simulink model "SOCPIControlBenchmark"  (R2019b)
settings: Solver=FixedStepAuto  StartTime=0.0  StopTime=30000  FixedStep=0.01  RelTol=1e-3
values from neighbouring files (symbols this model uses):
  kio = 0.6    [benchmarkPIDStart.m]
  kpo = 0.2    [benchmarkPIDStart.m]
  L = 0.1    [benchmarkPIDStart.m]
  maxKi = 0.1    [benchmarkPIDStart.m]
  maxKp = 0.1    [benchmarkPIDStart.m]
  minKi = 0.001    [benchmarkPIDStart.m]
  minKp = 0.01    [benchmarkPIDStart.m]
  N = 100    [benchmarkPIDStart.m]
  optimPeriod = 300    [benchmarkPIDStart.m]
  OVLim = 0.05    [benchmarkPIDStart.m]
  refSignalPeriod = 300    [benchmarkPIDStart.m]
  resetThreshold = 0.1    [benchmarkPIDStart.m]
  TSLim = 70    [benchmarkPIDStart.m]
undefined symbols (not defined in the file or in its folder): DiscIntNeverNeededParam
libraries: dspmathops x4, simulink x2
(part 1 of 3)
settings Model: Creator=jairo  LastModifiedBy=jairo
settings DataIOCC: ReturnWorkspaceOutputs=off

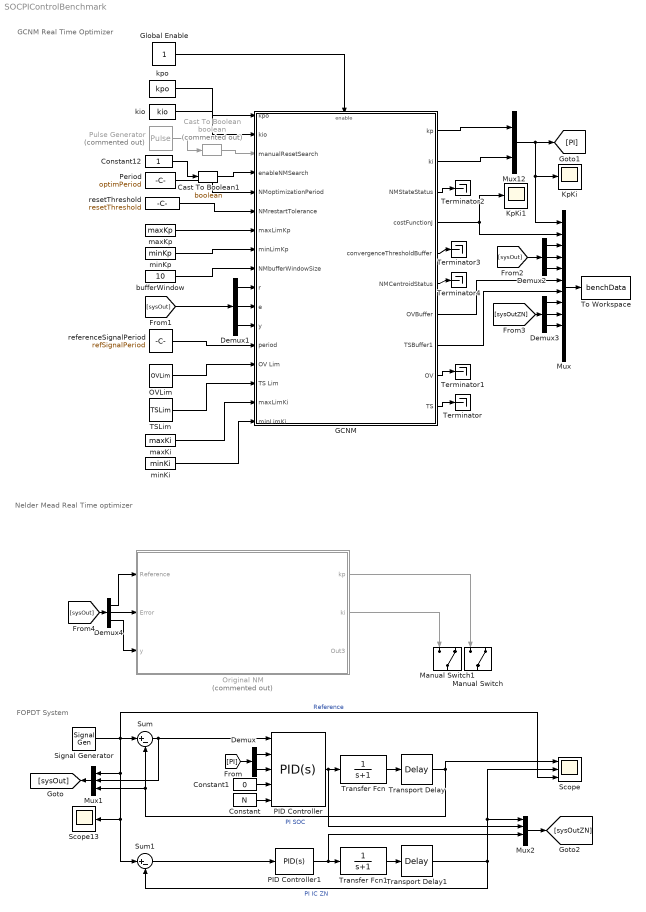
== system SOCPIControlBenchmark ==
  note: FOPDT System
  note: GCNM Real Time Optimizer
  note: Nelder Mead Real Time optimizer
  Cast To Boolean : DataTypeConversion  Commented=on  OutDataTypeStr=boolean
  Cast To Boolean1 : DataTypeConversion  OutDataTypeStr=boolean
  Constant : Constant  Value=N
  Constant1 : Constant  Value=0
  Constant12 : Constant  OutDataTypeStr=boolean
  Demux : Demux  Outputs=2
  Demux{1..4} (4 alike) : Demux  Outputs=3
  GCNM : Subsystem
  Global Enable : Constant
  KpKi : Scope
  KpKi1 : Scope
  Manual Switch : ManualSwitch  CurrentSetting=0
  Manual Switch1 : ManualSwitch  CurrentSetting=0
  Mux : Mux  Inputs=12
  Mux1 : Mux  Inputs=3
  Mux12 : Mux  Inputs=2
  Mux2 : Mux
  OVLim : Constant  Value=OVLim
  Original NM : Subsystem  Commented=on
  PID Controller : simulink/Continuous/PID Controller  Controller=PID  Form=Parallel  TimeDomain=Continuous-time  SampleTime=-1  IntegratorMethod=Forward Euler  FilterMethod=Forward Euler  ControllerParametersSource=external  P=1  I=100  D=0  UseFilter=on  N=100  TunerSelectOption=Transfer Function Based (PID Tuner App)  InitialConditionSource=internal  InitialConditionForIntegrator=0  InitialConditionForFilter=0  DifferentiatorICPrevScaledInput=0  ExternalReset=none  TrackingMode=off  Kt=1  LimitOutput=off  UpperSaturationLimit=inf  LowerSaturationLimit=-inf  LinearizeAsGain=on  AntiWindupMode=none  Kb=1  POutMin=[]  POutMax=[]  IOutMin=[]  IOutMax=[]  DOutMin=[]  DOutMax=[]  NOutMin=[]  NOutMax=[]  SumOutMin=[]  SumOutMax=[]  SaturationOutMin=[]  SaturationOutMax=[]  PParamMin=[]  PParamMax=[]  IParamMin=[]  IParamMax=[]  DParamMin=[]  DParamMax=[]  NParamMin=[]  NParamMax=[]  KbParamMin=[]  KbParamMax=[]  KtParamMin=[]  KtParamMax=[]  KbOutMin=[]  KbOutMax=[]  KtOutMin=[]  KtOutMax=[]  IntegratorOutMin=[]  IntegratorOutMax=[]  FilterOutMin=[]  FilterOutMax=[]  SumI1OutMin=[]  SumI1OutMax=[]  SumI2OutMin=[]  SumI2OutMax=[]  SumI3OutMin=[]  SumI3OutMax=[]  SumI4OutMin=[]  SumI4OutMax=[]  SumDOutMin=[]  SumDOutMax=[]  DifferentiatorOutMin=[]  DifferentiatorOutMax=[]  FilterDiffOutCoefMin=[]  FilterDiffOutCoefMax=[]  ReciprocalOutMin=[]  ReciprocalOutMax=[]  SumDenOutMin=[]  SumDenOutMax=[]  SumNumOutMin=[]  SumNumOutMax=[]  DivideOutMin=[]  DivideOutMax=[]  IntegratorContinuousStateAttributes=''  IntegratorStateMustResolveToSignalObject=off  IntegratorRTWStateStorageClass=Auto  FilterContinuousStateAttributes=''  FilterStateMustResolveToSignalObject=off  FilterRTWStateStorageClass=Auto  ParallelPVariant=ExternalParameters  IdealPVariant=Disabled  IVariant=ExternalParameters  DVariant=ExternalParameters  IntegratorVariant=Continuous  SatVariant=Disabled  AWVariant=Passthrough  PCopyVariant=Disabled  TRVariant=Disabled  FdbkBlocksVariant=Forward  IdealPFdbkVariant=Disabled  SatFdbkVariant=Disabled  DerivativeFilterVariant=ContFilter  NVariant=ExternalParameters  NCopyVariant=Disabled  FilterICVariant=InternalICsFilter  IntegratorICVariant=InternalICs  ExternalResetVariant=Disabled  TRSumVariant=Passthrough  SumFdbkVariant=Disabled  SumVariant=Sum_PID
  PID Controller1 : simulink/Continuous/PID Controller  Controller=PID  Form=Parallel  TimeDomain=Continuous-time  SampleTime=-1  IntegratorMethod=Forward Euler  FilterMethod=Forward Euler  ControllerParametersSource=internal  P=.12  I=0.006  D=0  UseFilter=on  N=100  TunerSelectOption=Transfer Function Based (PID Tuner App)  InitialConditionSource=internal  InitialConditionForIntegrator=0  InitialConditionForFilter=0  DifferentiatorICPrevScaledInput=0  ExternalReset=none  TrackingMode=off  Kt=1  LimitOutput=off  UpperSaturationLimit=inf  LowerSaturationLimit=-inf  LinearizeAsGain=on  AntiWindupMode=none  Kb=1  POutMin=[]  POutMax=[]  IOutMin=[]  IOutMax=[]  DOutMin=[]  DOutMax=[]  NOutMin=[]  NOutMax=[]  SumOutMin=[]  SumOutMax=[]  SaturationOutMin=[]  SaturationOutMax=[]  PParamMin=[]  PParamMax=[]  IParamMin=[]  IParamMax=[]  DParamMin=[]  DParamMax=[]  NParamMin=[]  NParamMax=[]  KbParamMin=[]  KbParamMax=[]  KtParamMin=[]  KtParamMax=[]  KbOutMin=[]  KbOutMax=[]  KtOutMin=[]  KtOutMax=[]  IntegratorOutMin=[]  IntegratorOutMax=[]  FilterOutMin=[]  FilterOutMax=[]  SumI1OutMin=[]  SumI1OutMax=[]  SumI2OutMin=[]  SumI2OutMax=[]  SumI3OutMin=[]  SumI3OutMax=[]  SumI4OutMin=[]  SumI4OutMax=[]  SumDOutMin=[]  SumDOutMax=[]  DifferentiatorOutMin=[]  DifferentiatorOutMax=[]  FilterDiffOutCoefMin=[]  FilterDiffOutCoefMax=[]  ReciprocalOutMin=[]  ReciprocalOutMax=[]  SumDenOutMin=[]  SumDenOutMax=[]  SumNumOutMin=[]  SumNumOutMax=[]  DivideOutMin=[]  DivideOutMax=[]  IntegratorContinuousStateAttributes=''  IntegratorStateMustResolveToSignalObject=off  IntegratorRTWStateStorageClass=Auto  FilterContinuousStateAttributes=''  FilterStateMustResolveToSignalObject=off  FilterRTWStateStorageClass=Auto  ParallelPVariant=InternalParameters  IdealPVariant=Disabled  IVariant=InternalParameters  DVariant=InternalParameters  IntegratorVariant=Continuous  SatVariant=Disabled  AWVariant=Passthrough  PCopyVariant=Disabled  TRVariant=Disabled  FdbkBlocksVariant=Forward  IdealPFdbkVariant=Disabled  SatFdbkVariant=Disabled  DerivativeFilterVariant=ContFilter  NVariant=InternalParameters  NCopyVariant=Disabled  FilterICVariant=InternalICsFilter  IntegratorICVariant=InternalICs  ExternalResetVariant=Disabled  TRSumVariant=Passthrough  SumFdbkVariant=Disabled  SumVariant=Sum_PID
  Period : Constant  Value=optimPeriod  OutDataTypeStr=double
  Pulse Generator : DiscretePulseGenerator  Commented=on  PulseType=Time based  Period=20  PulseWidth=0.1
  Scope : Scope  NumInputPorts=3
  Scope13 : Scope
  Signal Generator : SignalGenerator  WaveForm=square  Frequency=1/refSignalPeriod
  Sum : Sum  Inputs=|+-
  Sum1 : Sum  Inputs=|+-
  TSLim : Constant  Value=TSLim
  Terminator{,1..4} (5 alike) : Terminator
  To Workspace : ToWorkspace  VariableName=benchData  SaveFormat=Timeseries  SampleTime=-1
  Transfer Fcn : TransferFcn  Denominator=[1 1]
  Transfer Fcn1 : TransferFcn  Denominator=[1 1]
  Transport Delay : TransportDelay  DelayTime=L
  Transport Delay1 : TransportDelay  DelayTime=L
  bufferWindow : Constant  Value=10  OutDataTypeStr=uint16
  kio : Constant  Value=kio  OutDataTypeStr=double
  kpo : Constant  Value=kpo  OutDataTypeStr=double
  maxKi : Constant  Value=maxKi  VectorParams1D=off  OutDataTypeStr=double
  maxKp : Constant  Value=maxKp  OutDataTypeStr=double
  minKi : Constant  Value=minKi  OutDataTypeStr=double
  minKp : Constant  Value=minKp  OutDataTypeStr=double
  referenceSignalPeriod : Constant  Value=refSignalPeriod
  resetThreshold : Constant  Value=resetThreshold
  wires:
  PID Controller/1 -> Mux2/2, Transfer Fcn/1
  Transfer Fcn/1 -> Transport Delay/1
  Transfer Fcn1/1 -> Transport Delay1/1
  Sum1/1 -> PID Controller1/1
  PID Controller1/1 -> Mux2/3, Transfer Fcn1/1
  Sum/1 -> Mux1/2, PID Controller/1
  resetThreshold/1 -> GCNM/6(NMrestartTolerance)
  Mux12/1 -> Mux/1, KpKi/1, [PI]
  maxKp/1 -> GCNM/7(maxLimKp)
  bufferWindow/1 -> GCNM/9(NMbufferWindowSize)
  Cast To Boolean1/1 -> GCNM/4(enableNMSearch)
  kio/1 -> GCNM/2(kio)
  Pulse Generator/1 -> Cast To Boolean/1
  Cast To Boolean/1 -> GCNM/3(manualResetSearch)
  Constant12/1 -> Cast To Boolean1/1
  minKp/1 -> GCNM/8(minLimKp)
  Global Enable/1 -> GCNM/Enable
  kpo/1 -> GCNM/1(kpo)
  Period/1 -> GCNM/5(NMoptimizationPeriod)
  GCNM/4(costFunctionJ) -> Mux/2, KpKi1/1
  referenceSignalPeriod/1 -> GCNM/13("  period")
  OVLim/1 -> GCNM/14("  OV Lim")
  TSLim/1 -> GCNM/15(TS Lim)
  Transport Delay/1 -> Scope/1, Mux1/3, Sum/2  "PI SOC"
  Transport Delay1/1 -> Mux2/1, Scope/2, Sum1/2  "PI IC ZN"
  GCNM/1("  kp") -> Mux12/1
  GCNM/2("  ki") -> Mux12/2
  Original NM/1(kp) -> Manual Switch/1
  Original NM/2(ki) -> Manual Switch1/1
  Mux/1 -> To Workspace/1
  maxKi/1 -> GCNM/16(maxLimKi)
  minKi/1 -> GCNM/17(minLimKi)
  Constant/1 -> PID Controller/5
  Signal Generator/1 -> Sum1/1, Scope13/1, Mux1/1, Scope/3, Sum/1  "Reference"
  Constant1/1 -> PID Controller/4
  Demux/1 -> PID Controller/2
  Demux/2 -> PID Controller/3
  [PI] -> Demux/1
  Mux1/1 -> [sysOut]
  [sysOut] -> Demux1/1
  Demux1/1 -> GCNM/10("  r")
  Demux1/2 -> GCNM/11("  e")
  Demux1/3 -> GCNM/12("  y")
  [sysOut] -> Demux2/1
  Demux2/1 -> Mux/3
  Demux2/2 -> Mux/4
  Demux2/3 -> Mux/5
  Mux2/1 -> [sysOutZN]
  [sysOutZN] -> Demux3/1
  Demux3/1 -> Mux/8
  Demux3/2 -> Mux/9
  Demux3/3 -> Mux/10
  Demux4/2 -> Original NM/2(Error)
  Demux4/3 -> Original NM/3(y)
  [sysOut] -> Demux4/1
  Demux4/1 -> Original NM/1(Reference)
  GCNM/10(TS) -> Terminator/1
  GCNM/9(OV) -> Terminator1/1
  GCNM/8(TSBuffer1) -> Mux/7
  GCNM/7(OVBuffer) -> Mux/6
  GCNM/3(NMStateStatus) -> Terminator2/1
  GCNM/5(convergenceThresholdBuffer) -> Terminator3/1
  GCNM/6(NMCentroidStatus) -> Terminator4/1

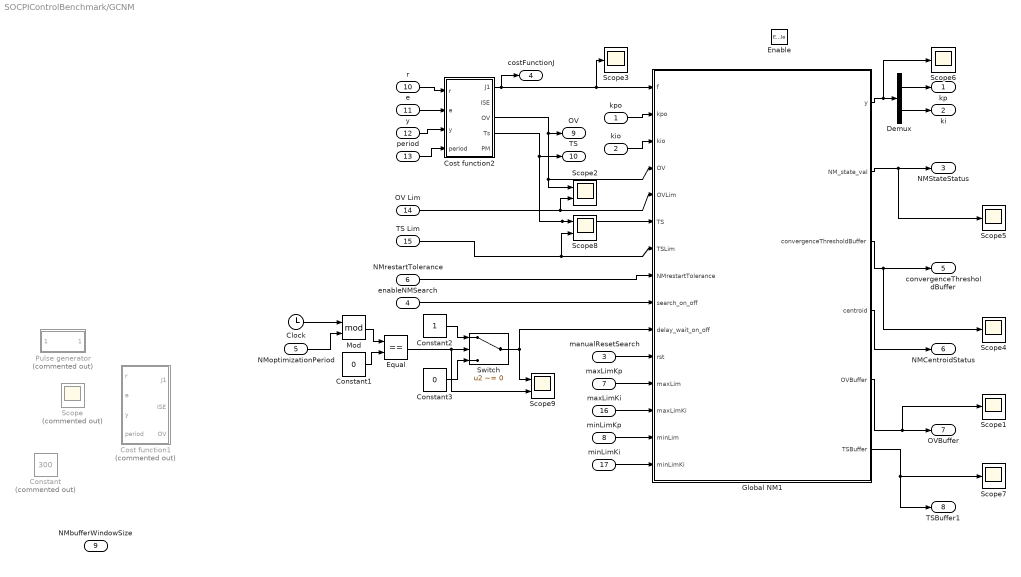
== system SOCPIControlBenchmark/GCNM ==
  kpo : Inport  OutDataTypeStr=double
  kio : Inport  Port=2  OutDataTypeStr=double
  manualResetSearch : Inport  Port=3  OutDataTypeStr=boolean
  enableNMSearch : Inport  Port=4  OutDataTypeStr=boolean
  NMoptimizationPeriod : Inport  Port=5  OutDataTypeStr=double
  NMrestartTolerance : Inport  Port=6
  maxLimKp : Inport  Port=7  OutDataTypeStr=double
  minLimKp : Inport  Port=8  OutDataTypeStr=double
  NMbufferWindowSize : Inport  Port=9  OutDataTypeStr=uint16
  "  r" : Inport  Port=10  OutDataTypeStr=double
  "  e" : Inport  Port=11  OutDataTypeStr=double
  "  y" : Inport  Port=12  OutDataTypeStr=double
  "  period" : Inport  Port=13  OutDataTypeStr=double
  "  OV Lim" : Inport  Port=14  OutDataTypeStr=double
  TS Lim : Inport  Port=15  OutDataTypeStr=double
  maxLimKi : Inport  Port=16  OutDataTypeStr=double
  minLimKi : Inport  Port=17  OutDataTypeStr=double
  Enable : EnablePort
  Clock : Clock
  Constant : Constant  Commented=on  Value=300
  Constant1 : Constant  Value=0
  Constant2 : Constant
  Constant3 : Constant  Value=0
  Cost function1 : Subsystem  Commented=on
  Cost function2 : Subsystem
  Demux : Demux  Outputs=2
  Equal : RelationalOperator  Operator===  RndMeth=Simplest
  Global NM1 : MATLAB Function  TreatAsAtomicUnit=on
  Mod : Math  Operator=mod  SignedPower=off  SaturateOnIntegerOverflow=on
  Pulse generator : Subsystem  Commented=on
  Scope : Scope  Commented=on
  Scope{1,3..7} (6 alike) : Scope
  Scope2 : Scope  NumInputPorts=2
  Scope8 : Scope  NumInputPorts=2
  Scope9 : Scope  NumInputPorts=2
  Switch : Switch  Criteria=u2 ~= 0
  "  kp" : Outport  OutDataTypeStr=double
  "  ki" : Outport  Port=2  OutDataTypeStr=double
  NMStateStatus : Outport  Port=3  OutDataTypeStr=double
  costFunctionJ : Outport  Port=4  OutDataTypeStr=double
  convergenceThresholdBuffer : Outport  Port=5  OutDataTypeStr=double
  NMCentroidStatus : Outport  Port=6  OutDataTypeStr=double
  OVBuffer : Outport  Port=7  OutDataTypeStr=double
  TSBuffer1 : Outport  Port=8  OutDataTypeStr=double
  OV : Outport  Port=9  OutDataTypeStr=double
  TS : Outport  Port=10  OutDataTypeStr=double
  wires:
  Demux/2 -> "  ki"/1
  Demux/1 -> "  kp"/1
  NMrestartTolerance/1 -> Global NM1/8(NMrestartTolerance)
  manualResetSearch/1 -> Global NM1/11(rst)
  enableNMSearch/1 -> Global NM1/9(search_on_off)
  minLimKp/1 -> Global NM1/14(minLim)
  maxLimKp/1 -> Global NM1/12(maxLim)
  Global NM1/2(NM_state_val) -> Scope5/1, NMStateStatus/1
  Global NM1/3(convergenceThresholdBuffer) -> convergenceThresholdBuffer/1, Scope4/1
  Global NM1/4(centroid) -> NMCentroidStatus/1
  Global NM1/1(y) -> Scope6/1, Demux/1
  kpo/1 -> Global NM1/2(kpo)
  kio/1 -> Global NM1/3(kio)
  Cost function2/3(OV) -> OV/1, Global NM1/4(OV), Scope2/1
  "  y"/1 -> Cost function2/3(y)
  "  e"/1 -> Cost function2/2(e)
  "  r"/1 -> Cost function2/1(r)
  Global NM1/5(OVBuffer) -> Scope1/1, OVBuffer/1
  "  period"/1 -> Cost function2/4(period)
  "  OV Lim"/1 -> Scope2/2, Global NM1/5(OVLim)
  Cost function2/4(Ts) -> TS/1, Global NM1/6(TS), Scope8/1
  TS Lim/1 -> Scope8/2, Global NM1/7(TSLim)
  Global NM1/6(TSBuffer) -> TSBuffer1/1, Scope7/1
  Cost function2/1(J1) -> Scope3/1, Global NM1/1(f), costFunctionJ/1
  Clock/1 -> Mod/1
  NMoptimizationPeriod/1 -> Mod/2
  Constant1/1 -> Equal/2
  Mod/1 -> Equal/1
  Constant2/1 -> Switch/1
  Constant3/1 -> Switch/3
  Switch/1 -> Scope9/1, Global NM1/10(delay_wait_on_off)
  Equal/1 -> Scope9/2, Switch/2
  maxLimKi/1 -> Global NM1/13(maxLimKi)
  minLimKi/1 -> Global NM1/15(minLimKi)

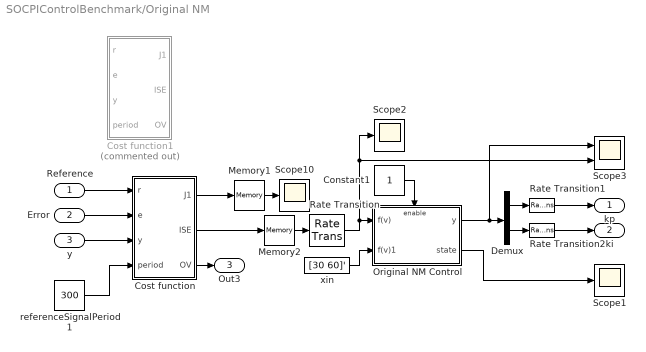
== system SOCPIControlBenchmark/Original NM ==
  Reference : Inport
  Error : Inport  Port=2
  y : Inport  Port=3
  Constant1 : Constant
  Cost function : Subsystem
  Cost function1 : Subsystem  Commented=on
  Demux : Demux  Outputs=2
  Memory1 : Memory
  Memory2 : Memory
  Original NM Control : Subsystem
  Rate Transition : RateTransition
  Rate Transition1 : RateTransition  InitialCondition=1
  Rate Transition2 : RateTransition  InitialCondition=100
  Scope1 : Scope
  Scope10 : Scope
  Scope2 : Scope
  Scope3 : Scope  NumInputPorts=2
  referenceSignalPeriod1 : Constant  Value=300
  xin : Constant  Value=[30 60]'
  kp : Outport
  ki : Outport  Port=2
  Out3 : Outport  Port=3
  wires:
  Constant1/1 -> Original NM Control/Enable
  Original NM Control/1(y) -> Scope3/1, Demux/1
  Rate Transition/1 -> Scope2/1, Scope3/2, Original NM Control/1(f(v))
  Demux/2 -> Rate Transition2/1
  xin/1 -> Original NM Control/2(f(v)1)
  y/1 -> Cost function/3(y)
  Original NM Control/2(state) -> Scope1/1
  Demux/1 -> Rate Transition1/1
  Memory2/1 -> Rate Transition/1
  Cost function/3(OV) -> Out3/1
  Memory1/1 -> Scope10/1
  referenceSignalPeriod1/1 -> Cost function/4(period)
  Cost function/1(J1) -> Memory1/1
  Cost function/2(ISE) -> Memory2/1
  Rate Transition1/1 -> kp/1
  Rate Transition2/1 -> ki/1
  Reference/1 -> Cost function/1(r)
  Error/1 -> Cost function/2(e)

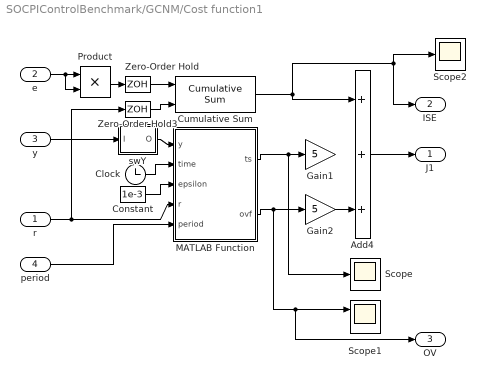
== system SOCPIControlBenchmark/GCNM/Cost function1 ==
  r : Inport
  e : Inport  Port=2
  y : Inport  Port=3
  period : Inport  Port=4
  Add4 : Sum  Inputs=+++
  Clock : Clock
  Constant : Constant  Value=1e-3
  Cumulative Sum : dspmathops/Cumulative Sum  dim=Channels (running sum)  InputProcessing=Columns as channels (frame based)  reset_popup=Falling edge  roundingMode=Floor  overflowMode=off  outputDataTypeStr=Inherit: Same as accumulator  outputMin=[]  outputMax=[]  outputLastDataTypeStr=Inherit: Same as accumulator
      settings: SourceProductName=DSP System Toolbox
  Gain1 : Gain  Gain=5
  Gain2 : Gain  Gain=5
  MATLAB Function : MATLAB Function  TreatAsAtomicUnit=on
  Product : Product
  Scope : Scope
  Scope1 : Scope  NumInputPorts=2
  Scope2 : Scope
  Zero-Order Hold : ZeroOrderHold  SampleTime=-1
  Zero-Order Hold3 : ZeroOrderHold  SampleTime=-1
  swY : Subsystem
  J1 : Outport
  ISE : Outport  Port=2
  OV : Outport  Port=3
  wires:
  period/1 -> MATLAB Function/5(period)
  Gain2/1 -> Add4/3
  Add4/1 -> J1/1
  y/1 -> swY/1(I)
  Constant/1 -> MATLAB Function/3(epsilon)
  Product/1 -> Zero-Order Hold/1
  Clock/1 -> MATLAB Function/2(time)
  swY/1(O) -> MATLAB Function/1(y)
  MATLAB Function/2(ovf) -> Gain2/1, Scope1/1, OV/1
  r/1 -> MATLAB Function/4(r), Zero-Order Hold3/1
  Zero-Order Hold/1 -> Cumulative Sum/1
  MATLAB Function/1(ts) -> Gain1/1, Scope/1
  e/1 -> Product/1, Product/2
  Zero-Order Hold3/1 -> Cumulative Sum/2
  Cumulative Sum/1 -> Scope2/1, ISE/1, Add4/1

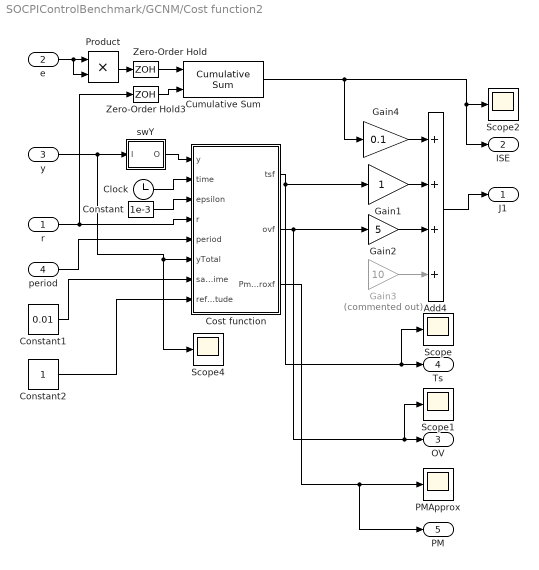
== system SOCPIControlBenchmark/GCNM/Cost function2 ==
  r : Inport
  e : Inport  Port=2
  y : Inport  Port=3
  period : Inport  Port=4
  Add4 : Sum  Inputs=++++
  Clock : Clock
  Constant : Constant  Value=1e-3
  Constant1 : Constant  Value=0.01
  Constant2 : Constant
  Cost function : MATLAB Function  TreatAsAtomicUnit=on
  Cumulative Sum : dspmathops/Cumulative Sum  dim=Channels (running sum)  InputProcessing=Columns as channels (frame based)  reset_popup=Falling edge  roundingMode=Floor  overflowMode=off  outputDataTypeStr=Inherit: Same as accumulator  outputMin=[]  outputMax=[]  outputLastDataTypeStr=Inherit: Same as accumulator
      settings: SourceProductName=DSP System Toolbox
  Gain1 : Gain
  Gain2 : Gain  Gain=5
  Gain3 : Gain  Commented=on  Gain=10
  Gain4 : Gain  Gain=0.1
  PMApprox : Scope
  Product : Product
  Scope{,1..2,4} (4 alike) : Scope
  Zero-Order Hold : ZeroOrderHold  SampleTime=-1
  Zero-Order Hold3 : ZeroOrderHold  SampleTime=-1
  swY : Subsystem
  J1 : Outport
  ISE : Outport  Port=2
  OV : Outport  Port=3
  Ts : Outport  Port=4
  PM : Outport  Port=5
  wires:
  Cumulative Sum/1 -> Gain4/1, ISE/1, Scope2/1
  Zero-Order Hold3/1 -> Cumulative Sum/2
  e/1 -> Product/2, Product/1
  Zero-Order Hold/1 -> Cumulative Sum/1
  r/1 -> Zero-Order Hold3/1, Cost function/4(r)
  swY/1(O) -> Cost function/1(y)
  Clock/1 -> Cost function/2(time)
  Product/1 -> Zero-Order Hold/1
  Constant/1 -> Cost function/3(epsilon)
  y/1 -> Scope4/1, Cost function/6(yTotal), swY/1(I)
  Add4/1 -> J1/1
  Gain2/1 -> Add4/3
  period/1 -> Cost function/5(period)
  Constant1/1 -> Cost function/7(samplingTime)
  Gain1/1 -> Add4/2
  Constant2/1 -> Cost function/8(refAmplitude)
  Gain3/1 -> Add4/4
  Cost function/1(tsf) -> Scope/1, Ts/1, Gain1/1
  Cost function/2(ovf) -> Scope1/1, OV/1, Gain2/1
  Cost function/3(PmAproxf) -> PM/1, PMApprox/1
  Gain4/1 -> Add4/1

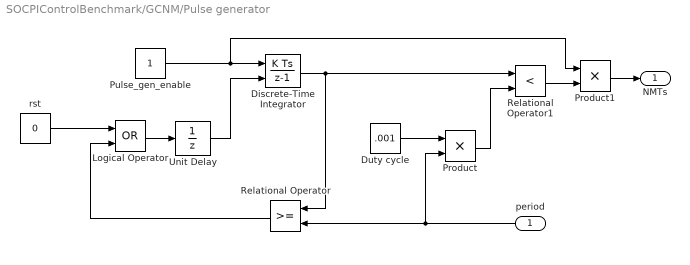
== system SOCPIControlBenchmark/GCNM/Pulse generator ==
  period : Inport
  Discrete-Time Integrator : DiscreteIntegrator  ExternalReset=rising  SampleTime=-1  ICPrevOutput=DiscIntNeverNeededParam  ICPrevScaledInput=DiscIntNeverNeededParam
  Duty cycle : Constant  Value=.001
  Logical Operator : Logic  Operator=OR  AllPortsSameDT=off  OutDataTypeStr=boolean
  Product : Product  RndMeth=Zero
  Product1 : Product  RndMeth=Zero
  Pulse_gen_enable : Constant
  Relational Operator : RelationalOperator  OutDataTypeStr=boolean  RndMeth=Nearest
  Relational Operator1 : RelationalOperator  Operator=<  OutDataTypeStr=boolean  RndMeth=Nearest
  Unit Delay : UnitDelay  SampleTime=-1
  rst : Constant  Value=0
  NMTs : Outport
  wires:
  Pulse_gen_enable/1 -> Discrete-Time Integrator/1, Product1/1
  Unit Delay/1 -> Discrete-Time Integrator/2
  Duty cycle/1 -> Product/1
  Product/1 -> Relational Operator1/2
  Discrete-Time Integrator/1 -> Relational Operator/1, Relational Operator1/1
  period/1 -> Relational Operator/2, Product/2
  Logical Operator/1 -> Unit Delay/1
  rst/1 -> Logical Operator/1
  Relational Operator/1 -> Logical Operator/2
  Relational Operator1/1 -> Product1/2
  Product1/1 -> NMTs/1

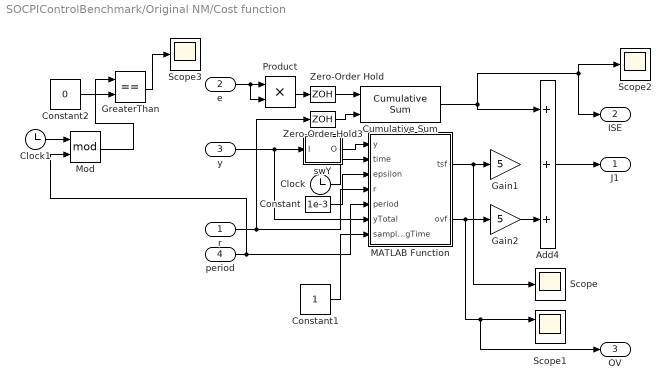
== system SOCPIControlBenchmark/Original NM/Cost function ==
  r : Inport
  e : Inport  Port=2
  y : Inport  Port=3
  period : Inport  Port=4
  Add4 : Sum  Inputs=+++
  Clock : Clock
  Clock1 : Clock
  Constant : Constant  Value=1e-3
  Constant1 : Constant
  Constant2 : Constant  Value=0
  Cumulative Sum : dspmathops/Cumulative Sum  dim=Channels (running sum)  InputProcessing=Columns as channels (frame based)  reset_popup=Falling edge  roundingMode=Floor  overflowMode=off  outputDataTypeStr=Inherit: Same as accumulator  outputMin=[]  outputMax=[]  outputLastDataTypeStr=Inherit: Same as accumulator
      settings: SourceProductName=DSP System Toolbox
  Gain1 : Gain  Gain=5
  Gain2 : Gain  Gain=5
  GreaterThan : RelationalOperator  Operator===  OutDataTypeStr=boolean  RndMeth=Simplest
  MATLAB Function : MATLAB Function  TreatAsAtomicUnit=on
  Mod : Math  Operator=mod  SignedPower=off  SaturateOnIntegerOverflow=on
  Product : Product
  Scope : Scope
  Scope1 : Scope  NumInputPorts=2
  Scope2 : Scope
  Scope3 : Scope
  Zero-Order Hold : ZeroOrderHold  SampleTime=-1
  Zero-Order Hold3 : ZeroOrderHold  SampleTime=-1
  swY : Subsystem
  J1 : Outport
  ISE : Outport  Port=2
  OV : Outport  Port=3
  wires:
  Cumulative Sum/1 -> Add4/1, ISE/1, Scope2/1
  Zero-Order Hold3/1 -> Cumulative Sum/2
  e/1 -> Product/2, Product/1
  MATLAB Function/1(tsf) -> Scope/1, Gain1/1
  Zero-Order Hold/1 -> Cumulative Sum/1
  r/1 -> Zero-Order Hold3/1, MATLAB Function/4(r)
  MATLAB Function/2(ovf) -> OV/1, Scope1/1, Gain2/1
  swY/1(O) -> MATLAB Function/1(y)
  Clock/1 -> MATLAB Function/2(time)
  Product/1 -> Zero-Order Hold/1
  Constant/1 -> MATLAB Function/3(epsilon)
  y/1 -> MATLAB Function/6(yTotal), swY/1(I)
  Add4/1 -> J1/1
  Gain2/1 -> Add4/3
  Constant1/1 -> MATLAB Function/7(samplingTime)
  Clock1/1 -> Mod/1
  Mod/1 -> GreaterThan/1
  period/1 -> MATLAB Function/5(period), Mod/2
  GreaterThan/1 -> Scope3/1
  Constant2/1 -> GreaterThan/2

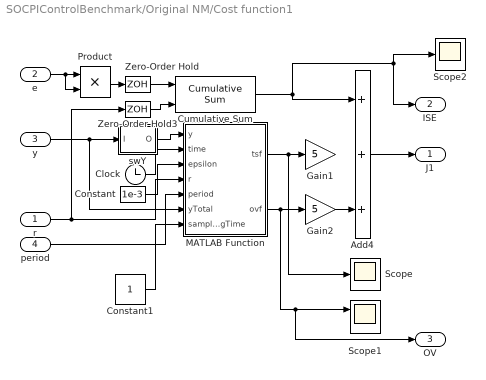
== system SOCPIControlBenchmark/Original NM/Cost function1 ==
  r : Inport
  e : Inport  Port=2
  y : Inport  Port=3
  period : Inport  Port=4
  Add4 : Sum  Inputs=+++
  Clock : Clock
  Constant : Constant  Value=1e-3
  Constant1 : Constant
  Cumulative Sum : dspmathops/Cumulative Sum  dim=Channels (running sum)  InputProcessing=Columns as channels (frame based)  reset_popup=Falling edge  roundingMode=Floor  overflowMode=off  outputDataTypeStr=Inherit: Same as accumulator  outputMin=[]  outputMax=[]  outputLastDataTypeStr=Inherit: Same as accumulator
      settings: SourceProductName=DSP System Toolbox
  Gain1 : Gain  Gain=5
  Gain2 : Gain  Gain=5
  MATLAB Function : MATLAB Function  TreatAsAtomicUnit=on
  Product : Product
  Scope : Scope
  Scope1 : Scope  NumInputPorts=2
  Scope2 : Scope
  Zero-Order Hold : ZeroOrderHold  SampleTime=-1
  Zero-Order Hold3 : ZeroOrderHold  SampleTime=-1
  swY : Subsystem
  J1 : Outport
  ISE : Outport  Port=2
  OV : Outport  Port=3
  wires:
  Constant1/1 -> MATLAB Function/7(samplingTime)
  period/1 -> MATLAB Function/5(period)
  Gain2/1 -> Add4/3
  Add4/1 -> J1/1
  y/1 -> swY/1(I), MATLAB Function/6(yTotal)
  Constant/1 -> MATLAB Function/3(epsilon)
  Product/1 -> Zero-Order Hold/1
  Clock/1 -> MATLAB Function/2(time)
  swY/1(O) -> MATLAB Function/1(y)
  MATLAB Function/2(ovf) -> Gain2/1, Scope1/1, OV/1
  r/1 -> MATLAB Function/4(r), Zero-Order Hold3/1
  Zero-Order Hold/1 -> Cumulative Sum/1
  MATLAB Function/1(tsf) -> Gain1/1, Scope/1
  e/1 -> Product/1, Product/2
  Zero-Order Hold3/1 -> Cumulative Sum/2
  Cumulative Sum/1 -> Scope2/1, ISE/1, Add4/1

== system SOCPIControlBenchmark/Original NM/Original NM Control ==
  note: Official backups
  f(v) : Inport
  f(v)1 : Inport  Port=2
  Enable : EnablePort
  Global NM : MATLAB Function  Commented=on  TreatAsAtomicUnit=on
  Original NM : MATLAB Function  Commented=on  TreatAsAtomicUnit=on
  Original NM2 : MATLAB Function  TreatAsAtomicUnit=on  SystemSampleTime=10
  Scope : Scope
  y : Outport
  state : Outport  Port=2
  wires:
  f(v)/1 -> Scope/1, Original NM2/1(f)
  Original NM2/1(y) -> y/1
  Original NM2/2(NM_state_val) -> state/1
  f(v)1/1 -> Original NM2/2(x)

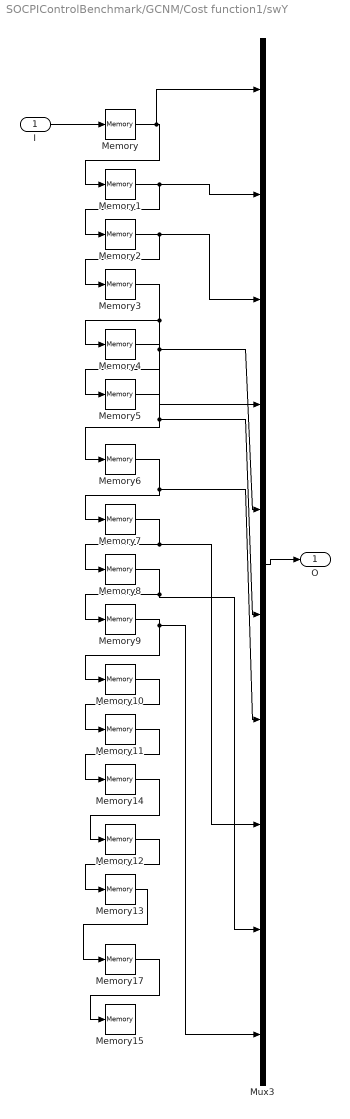
== system SOCPIControlBenchmark/GCNM/Cost function1/swY ==
  I : Inport
  Memory{,1..15,17} (17 alike) : Memory
  Mux3 : Mux  Inputs=10
  O : Outport
  wires:
  Memory17/1 -> Memory15/1
  Memory7/1 -> Mux3/8, Memory8/1
  Memory/1 -> Mux3/1, Memory1/1
  Memory8/1 -> Mux3/9, Memory9/1
  I/1 -> Memory/1
  Memory2/1 -> Mux3/3, Memory3/1
  Memory10/1 -> Memory11/1
  Memory1/1 -> Mux3/2, Memory2/1
  Memory6/1 -> Mux3/7, Memory7/1
  Memory3/1 -> Mux3/4, Memory4/1
  Memory9/1 -> Mux3/10, Memory10/1
  Mux3/1 -> O/1
  Memory4/1 -> Mux3/5, Memory5/1
  Memory5/1 -> Mux3/6, Memory6/1
  Memory13/1 -> Memory17/1
  Memory12/1 -> Memory13/1
  Memory14/1 -> Memory12/1
  Memory11/1 -> Memory14/1

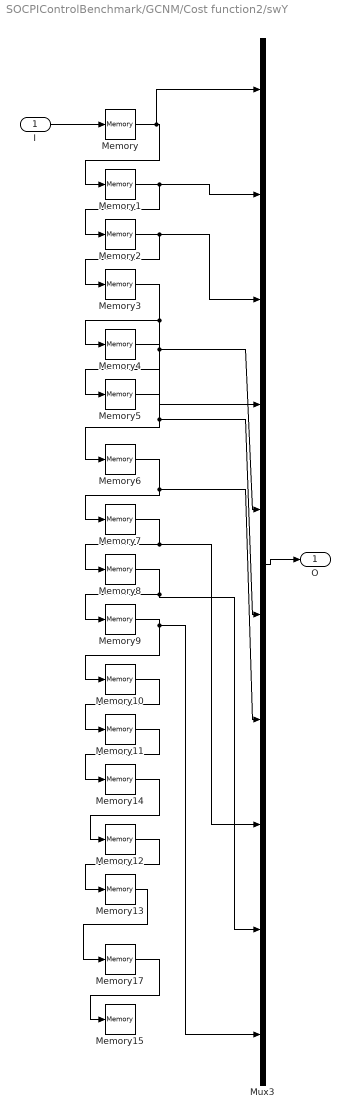
== system SOCPIControlBenchmark/GCNM/Cost function2/swY ==
  I : Inport
  Memory{,1..15,17} (17 alike) : Memory
  Mux3 : Mux  Inputs=10
  O : Outport
  wires:
  Memory11/1 -> Memory14/1
  Memory14/1 -> Memory12/1
  Memory12/1 -> Memory13/1
  Memory13/1 -> Memory17/1
  Memory5/1 -> Memory6/1, Mux3/6
  Memory4/1 -> Memory5/1, Mux3/5
  Mux3/1 -> O/1
  Memory9/1 -> Memory10/1, Mux3/10
  Memory3/1 -> Memory4/1, Mux3/4
  Memory6/1 -> Memory7/1, Mux3/7
  Memory1/1 -> Memory2/1, Mux3/2
  Memory10/1 -> Memory11/1
  Memory2/1 -> Memory3/1, Mux3/3
  I/1 -> Memory/1
  Memory8/1 -> Memory9/1, Mux3/9
  Memory/1 -> Memory1/1, Mux3/1
  Memory7/1 -> Memory8/1, Mux3/8
  Memory17/1 -> Memory15/1

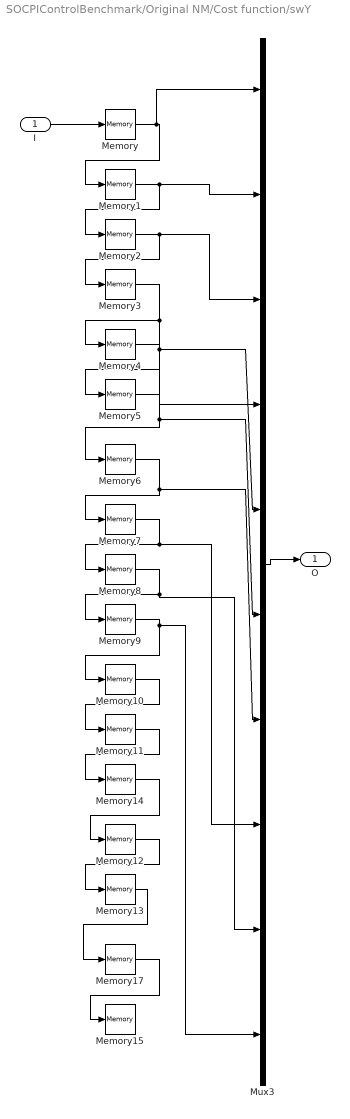
== system SOCPIControlBenchmark/Original NM/Cost function/swY ==
  I : Inport
  Memory{,1..15,17} (17 alike) : Memory
  Mux3 : Mux  Inputs=10
  O : Outport
  wires:
  Memory11/1 -> Memory14/1
  Memory14/1 -> Memory12/1
  Memory12/1 -> Memory13/1
  Memory13/1 -> Memory17/1
  Memory5/1 -> Memory6/1, Mux3/6
  Memory4/1 -> Memory5/1, Mux3/5
  Mux3/1 -> O/1
  Memory9/1 -> Memory10/1, Mux3/10
  Memory3/1 -> Memory4/1, Mux3/4
  Memory6/1 -> Memory7/1, Mux3/7
  Memory1/1 -> Memory2/1, Mux3/2
  Memory10/1 -> Memory11/1
  Memory2/1 -> Memory3/1, Mux3/3
  I/1 -> Memory/1
  Memory8/1 -> Memory9/1, Mux3/9
  Memory/1 -> Memory1/1, Mux3/1
  Memory7/1 -> Memory8/1, Mux3/8
  Memory17/1 -> Memory15/1

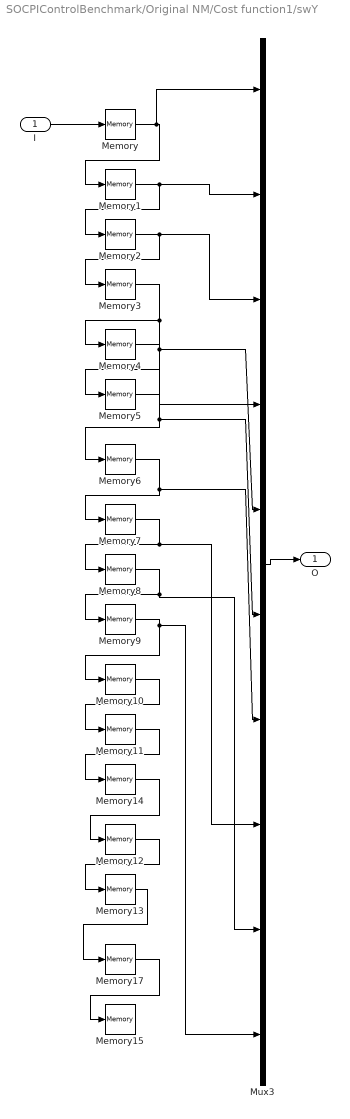
== system SOCPIControlBenchmark/Original NM/Cost function1/swY ==
  I : Inport
  Memory{,1..15,17} (17 alike) : Memory
  Mux3 : Mux  Inputs=10
  O : Outport
  wires:
  Memory17/1 -> Memory15/1
  Memory7/1 -> Mux3/8, Memory8/1
  Memory/1 -> Mux3/1, Memory1/1
  Memory8/1 -> Mux3/9, Memory9/1
  I/1 -> Memory/1
  Memory2/1 -> Mux3/3, Memory3/1
  Memory10/1 -> Memory11/1
  Memory1/1 -> Mux3/2, Memory2/1
  Memory6/1 -> Mux3/7, Memory7/1
  Memory3/1 -> Mux3/4, Memory4/1
  Memory9/1 -> Mux3/10, Memory10/1
  Mux3/1 -> O/1
  Memory4/1 -> Mux3/5, Memory5/1
  Memory5/1 -> Mux3/6, Memory6/1
  Memory13/1 -> Memory17/1
  Memory12/1 -> Memory13/1
  Memory14/1 -> Memory12/1
  Memory11/1 -> Memory14/1

== matlab function SOCPIControlBenchmark/Original NM/Cost function/MATLAB Function ==
  settings: updateMethod=DISCRETE
  data: y input; tsf output; time input; ovf output; epsilon input; r input; period input; yTotal input; samplingTime input
function [tsf,ovf] = performance(y,time,epsilon,r,period,yTotal,samplingTime)
        persistent OV tsFlag yHist counter ts;
        
        %initialization state
          if isempty(OV)        
              OV=0;
              tsFlag=1;
              yHist=zeros(1,round(period/(2*samplingTime)));
%               ts=0;
              counter=1;
              ts=0*samplingTime;
              tsf=0;
          end
          
          yHist(counter)=yTotal;
          
          %overshoot calculation
          OVCurrent=max(y);
          if OVCurrent>OV
              OV=OVCurrent;
              ovf=OV;
          else
              ovf=OV;
          end
          
          %calculate settling time each half of the period
          if mod(time,round(period/2))==0    
            ts=converTimeInv1s(yHist,10,epsilon);
%             yHist=zeros(1,round(period/2));
            counter=0;
            tsf=ts*samplingTime;
          else
              tsf=ts*samplingTime;
          end
          
          
          if mod(time,period)==0    %restart constraints after each repetitive period
            OV=0;
          end
          
          counter=counter+1;
          

end
